simulink model "SimpleBot_V1"  (R2024a)
settings: Solver=VariableStepAuto  StartTime=0.0  StopTime=1  FixedStep=0.01  RelTol=1e-3
PreLoadFcn:
  | run('Parameter.m')
values from neighbouring files (symbols this model uses):
  Achsabstand = 0.15    [Model1Sensibilities.m]    (also in Model1numericalPSA.m; Model2Sensibilities.m; Modellvalidierung.m; MotorSens2.m)
  Motoruebersetzung = 100    [Model1Sensibilities.m]    (also in Model1numericalPSA.m; Model2Sensibilities.m; Modellvalidierung.m; MotorSens2.m)
settings Model: Creator=jakob  LastModifiedBy=jakob

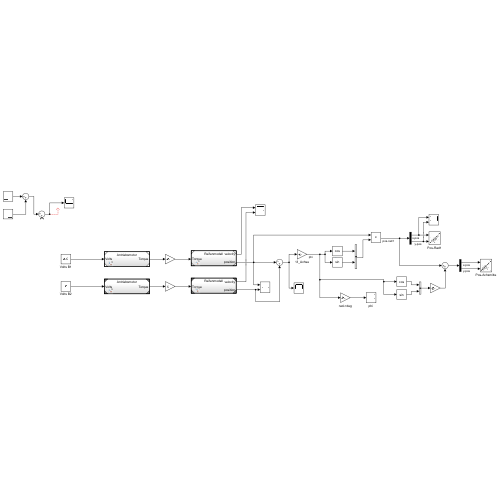
[thumbnail: Simulink's stored preview of the top-level diagram]
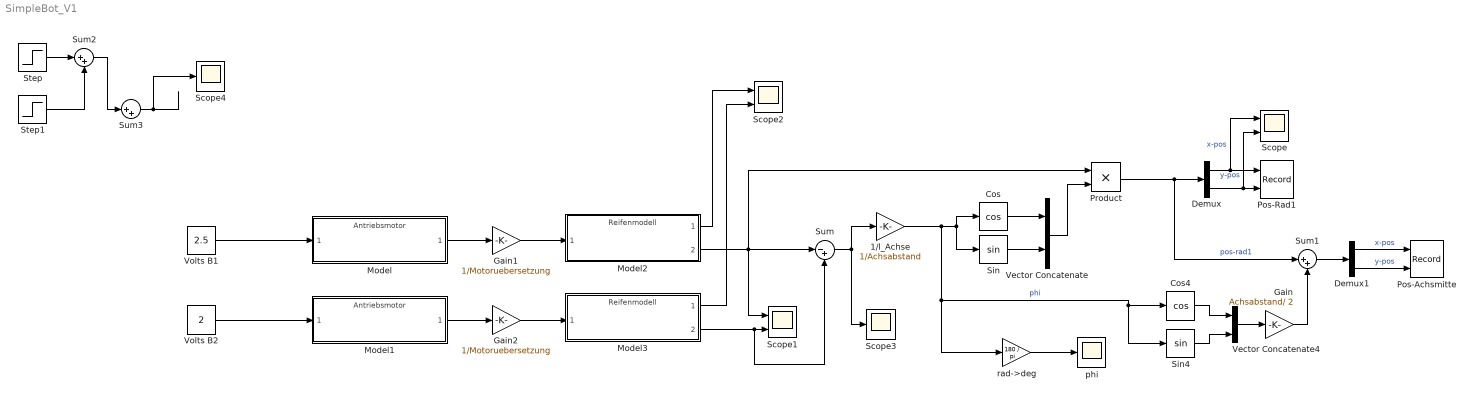
== system SimpleBot_V1 ==
  1/l_Achse : Gain  Gain=1/Achsabstand
  Cos : Trigonometry  Operator=cos
  Cos4 : Trigonometry  Operator=cos
  Demux : Demux  Outputs=2
  Demux1 : Demux  Outputs=2
  Gain : Gain  Gain=Achsabstand/ 2
  Gain1 : Gain  Gain=1/Motoruebersetzung
  Gain2 : Gain  Gain=1/Motoruebersetzung
  Model : ModelReference  ModelNameDialog=Antriebsmotor.slx  SimulationMode=Normal  ModelReferenceVersion=1.8
  Model1 : ModelReference  ModelNameDialog=Antriebsmotor.slx  SimulationMode=Normal  ModelReferenceVersion=1.8
  Model2 : ModelReference  ModelNameDialog=Reifenmodell.slx  SimulationMode=Normal  ModelReferenceVersion=1.10
  Model3 : ModelReference  ModelNameDialog=Reifenmodell.slx  SimulationMode=Normal  ModelReferenceVersion=1.10
  Pos-Achsmitte : Record  FileSettingsInternal="{\"entries\":[{\"content\":{\"excelSettings\":{\"content\":{},\"type\":\"Streamout.ExcelSettings\"}},\"type\":\"Streamout.FileSettingStorage\",\"uuid\":\"\"}],\"packageUris\":[\"http:\\/\\/schema.mathworks.com\\/mf0\\/streamout_blocks\\/R2020a\"],\"version\":\"1.0\"}"  Layout=[1 1]  SignalsInternal="{\"entries\":[{\"content\":{\"signals\":[{\"content\":{\"blockPath\":[],\"dimensions\":[1],\"domain\":\"\",\"lineColor\":\"#b746ff\",\"lineWidth\":2,\"plots\":[ 1 ],\"port\":1,\"sid\":[\"\"],\"signalID\":1,\"signalName\":\"x-pos\"},\"type\":\"RecordBlkView.Signal\",\"uuid\":\"\"},{\"content\":{\"blockPath\":[],\"dimensions\":[1],\"domain\":\"\",\"lineColor\":\"#139fff\",\"plots\":[ 1 ],\"port\":2,\"sid\":[\"\"],\"signalID\":2,\"signalName\":\"y-pos\"},\"type\":\"RecordBlkView.Signal\",\"uuid\":\"\"}]},\"type\":\"RecordBlkView.InputSignals\",\"uuid\":\"\"}],\"packageUris\":[\"http:\\/\\/schema.mathworks.com\\/mf0\\/streamout_blocks\\/R2020a\"],\"version\":\"1.0\"}"  VisualizationBindings="{\"xyplotplugin\":{\"info\":[{\"series\":[{\"bindingParametersList\":[{\"parameter\":\"X-Axis\",\"signalID\":1,\"signalName\":\"x-pos\"},{\"parameter\":\"Y-Axis\",\"signalID\":2,\"signalName\":\"y-pos\"}],\"seriesID\":0}],\"subplotID\":1}]}}"  CompatibilityTag=XY  st=-1
  Pos-Rad1 : Record  FileSettingsInternal="{\"entries\":[{\"content\":{\"excelSettings\":{\"content\":{},\"type\":\"Streamout.ExcelSettings\"}},\"type\":\"Streamout.FileSettingStorage\",\"uuid\":\"\"}],\"packageUris\":[\"http:\\/\\/schema.mathworks.com\\/mf0\\/streamout_blocks\\/R2020a\"],\"version\":\"1.0\"}"  Layout=[1 1]  SignalsInternal="{\"entries\":[{\"content\":{\"signals\":[{\"content\":{\"blockPath\":[],\"dimensions\":[1],\"domain\":\"\",\"lineColor\":\"#b746ff\",\"lineWidth\":2,\"plots\":[ 1 ],\"port\":1,\"sid\":[\"\"],\"signalID\":1,\"signalName\":\"x-pos\"},\"type\":\"RecordBlkView.Signal\",\"uuid\":\"\"},{\"content\":{\"blockPath\":[],\"dimensions\":[1],\"domain\":\"\",\"lineColor\":\"#139fff\",\"plots\":[ 1 ],\"port\":2,\"sid\":[\"\"],\"signalID\":2,\"signalName\":\"y-pos\"},\"type\":\"RecordBlkView.Signal\",\"uuid\":\"\"}]},\"type\":\"RecordBlkView.InputSignals\",\"uuid\":\"\"}],\"packageUris\":[\"http:\\/\\/schema.mathworks.com\\/mf0\\/streamout_blocks\\/R2020a\"],\"version\":\"1.0\"}"  VisualizationBindings="{\"xyplotplugin\":{\"info\":[{\"series\":[{\"bindingParametersList\":[{\"parameter\":\"X-Axis\",\"signalID\":1,\"signalName\":\"x-pos\"},{\"parameter\":\"Y-Axis\",\"signalID\":2,\"signalName\":\"y-pos\"}],\"seriesID\":0}],\"subplotID\":1}]}}"  CompatibilityTag=XY  st=-1
  Product : Product
  Scope : Scope  NumInputPorts=2
  Scope1 : Scope  NumInputPorts=2
  Scope2 : Scope  NumInputPorts=2
  Scope3 : Scope
  Scope4 : Scope
  Sin : Trigonometry
  Sin4 : Trigonometry
  Step : Step  Time=2  Before=2  After=6  SampleTime=0
  Step1 : Step  Time=3  Before=6  After=2  SampleTime=0
  Sum : Sum  Inputs=|-+
  Sum1 : Sum  Inputs=|++
  Sum2 : Sum  Inputs=|++
  Sum3 : Sum  Inputs=|++
  Vector Concatenate : Concatenate
  Vector Concatenate4 : Concatenate
  Volts B1 : Constant  Value=2.5
  Volts B2 : Constant  Value=2
  "phi " : Scope
  rad->deg : Gain  Gain=180 / pi
  wires:
  Model/1 -> Gain1/1
  Model1/1 -> Gain2/1
  Model3/2 -> Scope1/2, Sum/2
  Model2/2 -> Product/1, Sum/1, Scope1/1
  Sum/1 -> 1/l_Achse/1, Scope3/1
  Vector Concatenate/1 -> Product/2
  Cos/1 -> Vector Concatenate/1
  Sin/1 -> Vector Concatenate/2
  Product/1 -> Demux/1, Sum1/1  "pos-rad1"
  Demux/1 -> Scope/1, Pos-Rad1/1  "x-pos"
  Demux/2 -> Scope/2, Pos-Rad1/2  "y-pos"
  1/l_Achse/1 -> Sin/1, Cos/1, rad->deg/1, Cos4/1, Sin4/1  "phi"
  Model2/1 -> Scope2/1
  Model3/1 -> Scope2/2
  Volts B1/1 -> Model/1
  Volts B2/1 -> Model1/1
  rad->deg/1 -> "phi "/1
  Cos4/1 -> Vector Concatenate4/1
  Sin4/1 -> Vector Concatenate4/2
  Vector Concatenate4/1 -> Gain/1
  Gain/1 -> Sum1/2
  Sum1/1 -> Demux1/1
  Demux1/1 -> Pos-Achsmitte/1  "x-pos"
  Demux1/2 -> Pos-Achsmitte/2  "y-pos"
  Gain1/1 -> Model2/1
  Gain2/1 -> Model3/1
  Step/1 -> Sum2/1
  Step1/1 -> Sum2/2
  Sum2/1 -> Sum3/1
  Sum3/1 -> Scope4/1
